simulink model "Grid_PV_three_phase"  (R2024a)
settings: Solver=VariableStepAuto  StartTime=0.0  StopTime=2.0  RelTol=1e-3
libraries: spsSeriesRLCBranchLib x12, spsIGBTDiodeLib x7, slpidlib x5, spsCurrentMeasurementLib x3, spsAlphaBetaZerotodq0Lib x3, simulink x2, spsabctoAlphaBetaZeroLib x2, spsThreePhaseVIMeasurementLib x2, spsPVArrayLib x1, spsDiodeLib x1, spsMeanLib x1, spsdq0toabcLib x1
settings Model: Creator=Ashmita  LastModifiedBy=Ashmita

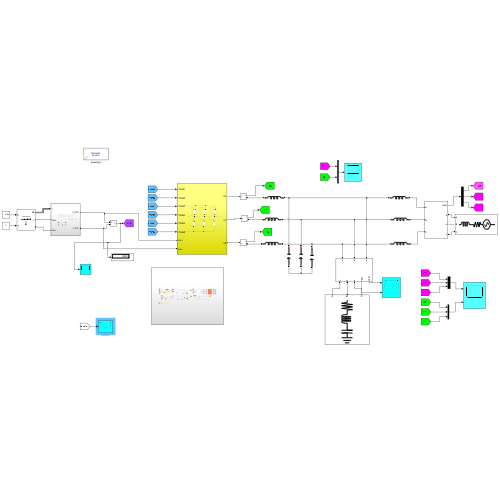
[thumbnail: Simulink's stored preview of the top-level diagram]
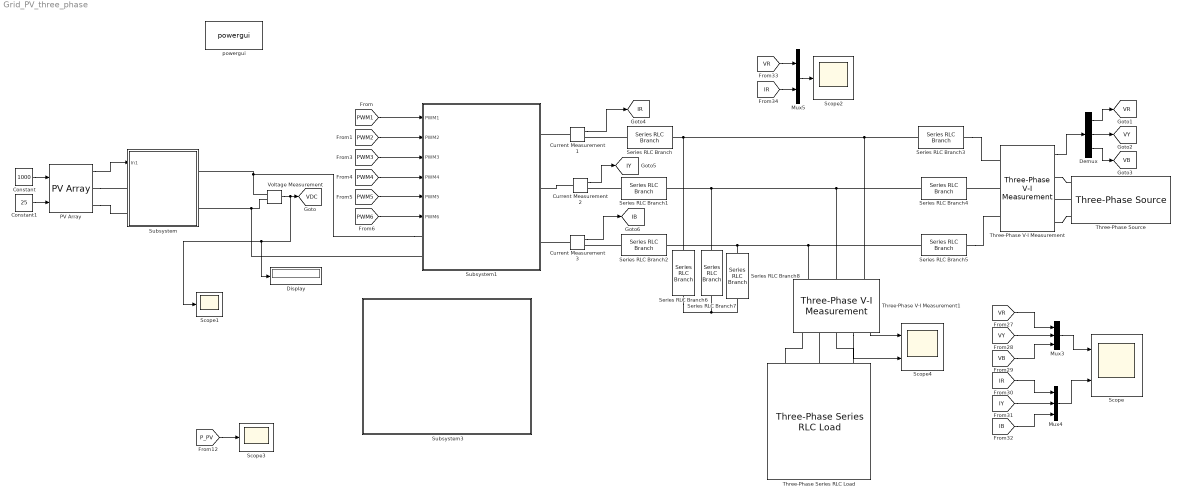
== system Grid_PV_three_phase ==
  Constant : Constant  Value=1000
  Constant1 : Constant  Value=25
  Current Measurement1 : spsCurrentMeasurementLib/Current Measurement  PhasorSimulation=off  OutputType=Complex  PSBequivalent=0
  Current Measurement2 : spsCurrentMeasurementLib/Current Measurement  PhasorSimulation=off  OutputType=Complex  PSBequivalent=0
  Current Measurement3 : spsCurrentMeasurementLib/Current Measurement  PhasorSimulation=off  OutputType=Complex  PSBequivalent=0
  Demux : Demux  Outputs=3
  Display : Display
  Mux3 : Mux  Inputs=3
  Mux4 : Mux  Inputs=3
  Mux5 : Mux  Inputs=2
  PV Array : spsPVArrayLib/PV Array  Npar=40  Nser=20  PlotType=array @ 1000 W/m2 & specified temperatures  S_vec="[ 1000  500  100 ]"  Temp_C_vec="[ 45 25  ]"  ModuleName=User-defined  PlotWhenSelected=off  Pm=213.15  Ncell=60  Voc=36.3  Isc=7.84  Vm=29  Im=7.35  beta_Voc_pc=-0.36099  alpha_Isc_pc=0.102  beta_Voc=-0.13104  alpha_Isc=0.0079968  IL=7.8654  I0=2.9273e-10  nI=0.98119  Rsh=313.0553  Rs=0.39381  RobustModel=off  RobustCellTemperature=313.3991  BAL=on  Tc=1e-6  Tfilter=5e-5
  Scope : Scope  NumInputPorts=2
  Scope1 : Scope
  Scope2 : Scope
  Scope3 : Scope
  Scope4 : Scope  NumInputPorts=2
  Series RLC Branch{,1..5} (6 alike) : spsSeriesRLCBranchLib/Series RLC Branch  LConnTagsString=__new0  RConnTagsString=__new0  BranchType=L  Resistance=1  Inductance=500e-6  SetiL0=off  InitialCurrent=0  Capacitance=1e-6  Setx0=off  InitialVoltage=0  Measurements=None
  Series RLC Branch6 : spsSeriesRLCBranchLib/Series RLC Branch  LConnTagsString=__new0  RConnTagsString=__new0  BranchType=C  Resistance=1  Inductance=500e-6  SetiL0=off  InitialCurrent=0  Capacitance=100e-6  Setx0=off  InitialVoltage=0  Measurements=None
  Series RLC Branch7 : spsSeriesRLCBranchLib/Series RLC Branch  LConnTagsString=__new0  RConnTagsString=__new0  BranchType=C  Resistance=1  Inductance=500e-6  SetiL0=off  InitialCurrent=0  Capacitance=100e-6  Setx0=off  InitialVoltage=0  Measurements=None
  Series RLC Branch8 : spsSeriesRLCBranchLib/Series RLC Branch  LConnTagsString=__new0  RConnTagsString=__new0  BranchType=C  Resistance=1  Inductance=500e-6  SetiL0=off  InitialCurrent=0  Capacitance=100e-6  Setx0=off  InitialVoltage=0  Measurements=None
  Subsystem : Subsystem
  Subsystem1 : Subsystem
  Subsystem3 : Subsystem
  Three-Phase Series RLC Load : spsThreePhaseSeriesRLCLoadLib/Three-Phase Series RLC Load  LConnTagsString=A|B|C  Configuration=Y (grounded)  NominalVoltage=1000  Vabc=[1e3 1e3 1e3]  Vabcp=[1e3 1e3 1e3]  NominalFrequency=60  UnbalancedPower=off  ActivePower=10e3  InductivePower=100  CapacitivePower=100  Pabc=[10e3 9e3 11e3]  QLabc=[100 90 110]  QCabc=[100 90 110]  Pabcp=[10e3 9e3 11e3]  QLabcp=[100 90 110]  QCabcp=[100 90 110]  Measurements=None  LoadType=constant Z
  Three-Phase V-I Measurement : spsThreePhaseVIMeasurementLib/Three-Phase V-I Measurement  VoltageMeasurement=phase-to-phase  SetLabelV=off  LabelV=Vabc  Vpu=off  VpuLL=off  CurrentMeasurement=no  SetLabelI=off  LabelI=Iabc  Ipu=off  Pbase=100e6  Vbase=500e3  OutputType=Complex  PhasorSimulation=off  PSBequivalent=0
  Three-Phase V-I Measurement1 : spsThreePhaseVIMeasurementLib/Three-Phase V-I Measurement  VoltageMeasurement=phase-to-phase  SetLabelV=off  LabelV=Vabc  Vpu=off  VpuLL=off  CurrentMeasurement=yes  SetLabelI=off  LabelI=Iabc  Ipu=off  Pbase=100e6  Vbase=500e3  OutputType=Complex  PhasorSimulation=off  PSBequivalent=0
  Three-Phase Source : spsThreePhaseSourceLib/Three-Phase Source  InternalConnection=Y  VoltagePhases=off  Voltage=415  PhaseAngle=0  Voltage_phases=[25e3 25e3 25e3]/sqrt(3)  PhaseAngles_phases=[0 -120 +120]  Frequency=50  NonIdealSource=on  SpecifyImpedance=off  Resistance=0.001e-3  Inductance=0.001e-9  ShortCircuitLevel=100e6  BaseVoltage=415  XRratio=7  BusType=swing  Pref=10e3  Qref=0  Prefabc=[10e3, 10e3, 10e3]  Qrefabc=[0, 0, 0]  Qmin=-inf  Qmax=inf
  Voltage Measurement : spsVoltageMeasurementLib/Voltage Measurement  PhasorSimulation=off  OutputType=Complex  PSBequivalent=0
  powergui : sps_lib/powergui  Priority=1  SimulationMode=Discrete  SampleTime=1e-6  frequency=60  Iterations=50  frequencyindice=50  Pbase=100e6  ErrMax=1e-4  UnitsV=kV  UnitsW=MW  buscounter=0  FunctionMessages=off  echomessages=off  EnableUseOfTLC=off  CurrentSourceSwitches=off  DisableSnubberDevices=off  DisableRonSwitches=off  DisableVfSwitches=off  DisplayEquations=off  AutomaticDiscreteSolvers=off  SolverType=Tustin/Backward Euler (TBE)  Interpol=off  ExternalGateDelay=off  methode=off  Ts=100  x0status=blocks  SPID=on  SwTol=0  HookPort=off  NonlinearTolerance=0  nMaxIteration=15  ContinueOnMaxIteration=off  RestoreLinks=warning  ResistiveCurrentMeasurement=off  Frange=[0:2:500]  Ylog=off  Xlog=on  ShowGrid=off  save=off  variable=ZData  structure=grid  ZoomFFT=on  StartTime=0.01  cycles=4  DisplayStyle=1  fundamental=50  FreqAxis=on  MaxFrequency=1000  frequencyindicesteady=1  RmsSteady=1  display=off
  tag scope: IB=global, IR=global, IY=global, VB=global, VDC=global, VR=global, VY=global
  wires:
  Constant1/1 -> PV Array/2
  PV Array/1 -> Subsystem/1(In1)
  Constant/1 -> PV Array/1
  Mux3/1 -> Scope/1
  [IR] -> Mux5/2
  [PWM6] -> Subsystem1/6("\tPWM6")
  [IR] -> Mux4/1
  [VR] -> Mux5/1
  [IY] -> Mux4/2
  [VB] -> Mux3/3
  [VY] -> Mux3/2
  [VR] -> Mux3/1
  [PWM3] -> Subsystem1/3("\tPWM3")
  [IB] -> Mux4/3
  Three-Phase V-I Measurement/1 -> Demux/1
  [PWM4] -> Subsystem1/4("\tPWM4")
  Current Measurement2/1 -> [IY]
  Mux4/1 -> Scope/2
  Demux/2 -> [VY]
  Demux/1 -> [VR]
  Demux/3 -> [VB]
  Current Measurement3/1 -> [IB]
  [PWM5] -> Subsystem1/5("\tPWM5")
  [PWM1] -> Subsystem1/1("\tPWM1 ")
  [PWM2] -> Subsystem1/2("\tPWM2")
  Current Measurement1/1 -> [IR]
  Mux5/1 -> Scope2/1
  Voltage Measurement/1 -> Display/1, Scope1/1, [VDC]
  Three-Phase V-I Measurement1/1 -> Scope4/1
  Three-Phase V-I Measurement1/2 -> Scope4/2
  [P_PV] -> Scope3/1
  connections:
  Voltage Measurement/LConn2 -- Subsystem1/LConn2 -- Subsystem/RConn2
  PV Array/RConn2 -- Subsystem/LConn2
  PV Array/RConn1 -- Subsystem/LConn1
  Subsystem1/LConn1 -- Subsystem/RConn1 -- Voltage Measurement/LConn1
  Series RLC Branch8/LConn1 -- Three-Phase V-I Measurement1/LConn3 -- Series RLC Branch5/LConn1 -- Series RLC Branch2/RConn1
  Series RLC Branch8/RConn1 -- Series RLC Branch6/RConn1 -- Series RLC Branch7/RConn1
  Series RLC Branch/RConn1 -- Three-Phase V-I Measurement1/LConn1 -- Series RLC Branch3/LConn1 -- Series RLC Branch6/LConn1
  Series RLC Branch1/RConn1 -- Three-Phase V-I Measurement1/LConn2 -- Series RLC Branch4/LConn1 -- Series RLC Branch7/LConn1
  Series RLC Branch2/LConn1 -- Current Measurement3/RConn1
  Series RLC Branch3/RConn1 -- Three-Phase V-I Measurement/LConn1
  Three-Phase Source/RConn2 -- Three-Phase V-I Measurement/RConn2
  Series RLC Branch/LConn1 -- Current Measurement1/RConn1
  Series RLC Branch1/LConn1 -- Current Measurement2/RConn1
  Current Measurement2/LConn1 -- Subsystem1/RConn2
  Three-Phase V-I Measurement/RConn1 -- Three-Phase Source/RConn1
  Series RLC Branch5/RConn1 -- Three-Phase V-I Measurement/LConn3
  Three-Phase V-I Measurement/LConn2 -- Series RLC Branch4/RConn1
  Current Measurement3/LConn1 -- Subsystem1/RConn3
  Three-Phase V-I Measurement/RConn3 -- Three-Phase Source/RConn3
  Current Measurement1/LConn1 -- Subsystem1/RConn1
  Three-Phase Series RLC Load/LConn1 -- Three-Phase V-I Measurement1/RConn3
  Three-Phase Series RLC Load/LConn2 -- Three-Phase V-I Measurement1/RConn2
  Three-Phase Series RLC Load/LConn3 -- Three-Phase V-I Measurement1/RConn1

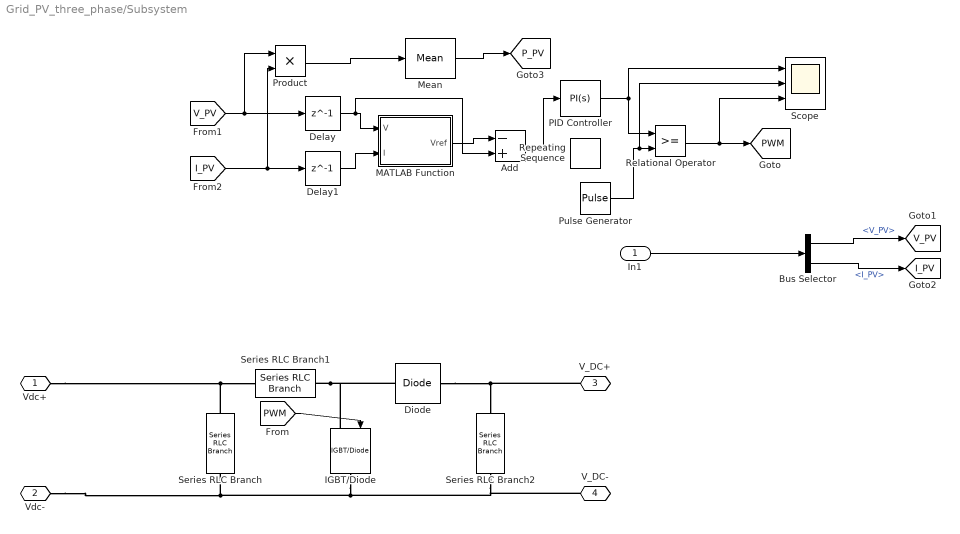
== system Grid_PV_three_phase/Subsystem ==
  In1 : Inport
  Add : Sum  Inputs=-+
  Bus Selector : BusSelector  OutputSignals=V_PV,I_PV
  Delay : Delay  DelayLength=1  InitialCondition=0
  Delay1 : Delay  DelayLength=1  InitialCondition=0
  Diode : spsDiodeLib/Diode  Ron=0.001  Lon=2.2e-3  Vf=0.7  IC=0  UseSnubber=0  Rs=10e3  Cs=inf  Measurements=off
  IGBT/Diode : spsIGBTDiodeLib/IGBT//Diode  Ron=.001  Rs=1e3  Cs=inf  Measurements=off
  MATLAB Function : MATLAB Function  TreatAsAtomicUnit=on
  Mean : spsMeanLib/Mean  Freq=60  Vinit=0  Ts=0
  PID Controller : slpidlib/PID Controller  Controller=PI  Form=Parallel  TimeDomain=Continuous-time  UseExternalTs=off  SampleTime=-1  IntegratorMethod=Forward Euler  FilterMethod=Forward Euler  ControllerParametersSource=internal  P=0.05  I=0.01  UseKiTs=off  D=0  UseExternalDerivativeSource=off  N=100  UseFilter=on  TunerSelectOption=Transfer Function Based (PID Tuner App)  InitialConditionSource=internal  InitialConditionForIntegrator=0  InitialConditionForFilter=0  DifferentiatorICPrevScaledInput=0  ExternalReset=none  TrackingMode=off  Kt=1  LimitOutput=on  SatLimitsSource=internal  UpperSaturationLimit=0.95  LowerSaturationLimit=0.00  LinearizeAsGain=on  AntiWindupMode=none  Kb=1  LimitIntegrator=off  UpperIntegratorSaturationLimit=inf  LowerIntegratorSaturationLimit=-inf  POutMin=[]  POutMax=[]  IOutMin=[]  IOutMax=[]  DOutMin=[]  DOutMax=[]  NOutMin=[]  NOutMax=[]  SumOutMin=[]  SumOutMax=[]  SaturationOutMin=[]  SaturationOutMax=[]  PParamMin=[]  PParamMax=[]  IParamMin=[]  IParamMax=[]  DParamMin=[]  DParamMax=[]  NParamMin=[]  NParamMax=[]  KbParamMin=[]  KbParamMax=[]  KtParamMin=[]  KtParamMax=[]  KbOutMin=[]  KbOutMax=[]  KtOutMin=[]  KtOutMax=[]  IntegratorOutMin=[]  IntegratorOutMax=[]  FilterOutMin=[]  FilterOutMax=[]  SumI1OutMin=[]  SumI1OutMax=[]  SumI2OutMin=[]  SumI2OutMax=[]  SumI3OutMin=[]  SumI3OutMax=[]  SumI4OutMin=[]  SumI4OutMax=[]  SumDOutMin=[]  SumDOutMax=[]  DifferentiatorOutMin=[]  DifferentiatorOutMax=[]  FilterDiffOutCoefMin=[]  FilterDiffOutCoefMax=[]  ReciprocalOutMin=[]  ReciprocalOutMax=[]  SumDenOutMin=[]  SumDenOutMax=[]  SumNumOutMin=[]  SumNumOutMax=[]  DivideOutMin=[]  DivideOutMax=[]  UdiffTsProdOutMin=[]  UdiffTsProdOutMax=[]  NTsProdOutMin=[]  NTsProdOutMax=[]  UintegralTsProdOutMin=[]  UintegralTsProdOutMax=[]  UngainTsProdOutMin=[]  UngainTsProdOutMax=[]  ClampingZeroOutDataTypeStr=Inherit: Inherit via back propagation  ClampingZeroOutMin=[]  ClampingZeroOutMax=[]  FilterDenConstantOutDataTypeStr=Inherit: Inherit via back propagation  FilterDenConstantOutMin=[]  FilterDenConstantOutMax=[]  PCopyOutDataTypeStr=Inherit: Inherit via back propagation  PCopyOutMin=[]  PCopyOutMax=[]  NCopyOutDataTypeStr=Inherit: Inherit via back propagation  NCopyOutMin=[]  NCopyOutMax=[]  IntegratorContinuousStateAttributes=''  IntegratorStateMustResolveToSignalObject=off  IntegratorRTWStateStorageClass=Auto  FilterContinuousStateAttributes=''  FilterStateMustResolveToSignalObject=off  FilterRTWStateStorageClass=Auto  ParallelPVariant=InternalParameters  IdealPVariant=Disabled  IVariant=InternalParameters  DVariant=Disabled  IntegratorVariant=Continuous  SatVariant=Enabled  AWVariant=Passthrough  PCopyVariant=Disabled  TRVariant=Disabled  FdbkBlocksVariant=Forward  IdealPFdbkVariant=Disabled  SatFdbkVariant=Disabled  DerivativeFilterVariant=Disabled  NVariant=Disabled  NCopyVariant=Disabled_SignalSpec  FilterICVariant=Disabled  IntegratorICVariant=InternalICs  ExternalResetVariant=Disabled  TRSumVariant=Passthrough  SumFdbkVariant=Disabled  SumVariant=Sum_PI  TsampFilterVariant=InternalTs  TsampNgainVariant=Passthrough  TsampIntegralVariant=Disabled_SignalSpec  ExternalSaturationOutDataTypeStr=Inherit: Same as second input  DerivativeSourceVariant=Disabled
  Product : Product
  Pulse Generator : DiscretePulseGenerator  PulseType=Time based  Period=1/500000  PulseWidth=90
  Relational Operator : RelationalOperator  OutDataTypeStr=boolean  RndMeth=Simplest  InputSameDT=off
  Repeating Sequence : simulink/Sources/Repeating Sequence  rep_seq_t=[0 1/5000]  rep_seq_y=[0 1]
  Scope : Scope  NumInputPorts=3
  Series RLC Branch : spsSeriesRLCBranchLib/Series RLC Branch  LConnTagsString=__new0  RConnTagsString=__new0  BranchType=C  Resistance=1e-6  Inductance=1e-3  SetiL0=off  InitialCurrent=0  Capacitance=1000e-6  Setx0=off  InitialVoltage=0  Measurements=None
  Series RLC Branch1 : spsSeriesRLCBranchLib/Series RLC Branch  LConnTagsString=__new0  RConnTagsString=__new0  BranchType=L  Resistance=1  Inductance=1.45e-3  SetiL0=off  InitialCurrent=0  Capacitance=1e-6  Setx0=off  InitialVoltage=0  Measurements=None
  Series RLC Branch2 : spsSeriesRLCBranchLib/Series RLC Branch  LConnTagsString=__new0  RConnTagsString=__new0  BranchType=C  Resistance=1  Inductance=1e-3  SetiL0=off  InitialCurrent=0  Capacitance=3227e-6  Setx0=off  InitialVoltage=0  Measurements=None
  Vdc+ : PMIOPort  Side=Left
  V_DC+ : PMIOPort  Port=3  Side=Right
  V_DC- : PMIOPort  Port=4  Side=Right
  Vdc- : PMIOPort  Port=2  Side=Left
  tag scope: I_PV=global, PWM=global, P_PV=global, V_PV=global
  wires:
  [V_PV] -> Product/1, Delay/1
  [I_PV] -> Product/2, Delay1/1
  Mean/1 -> [P_PV]
  Add/1 -> PID Controller/1
  Delay/1 -> Add/2, MATLAB Function/1(V)
  Product/1 -> Mean/1
  Bus Selector/1 -> [V_PV]  "<V_PV>"
  MATLAB Function/1(Vref) -> Add/1
  PID Controller/1 -> Relational Operator/1, Scope/1
  Relational Operator/1 -> Scope/3, [PWM]
  Delay1/1 -> MATLAB Function/2(I)
  Bus Selector/2 -> [I_PV]  "<I_PV>"
  [PWM] -> IGBT/Diode/1
  In1/1 -> Bus Selector/1
  Pulse Generator/1 -> Scope/2, Relational Operator/2
  connections:
  Diode/RConn1 -- V_DC+/RConn1 -- Series RLC Branch2/LConn1
  Series RLC Branch1/LConn1 -- IGBT/Diode/LConn1 -- Diode/LConn1
  IGBT/Diode/RConn1 -- V_DC-/RConn1 -- Series RLC Branch2/RConn1 -- Vdc-/RConn1 -- Series RLC Branch/RConn1
  Series RLC Branch/LConn1 -- Vdc+/RConn1 -- Series RLC Branch1/RConn1

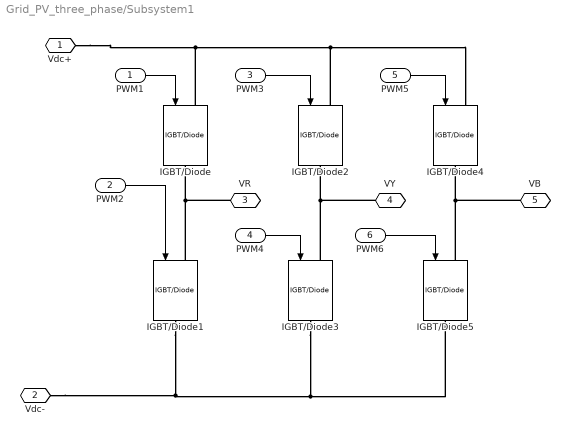
== system Grid_PV_three_phase/Subsystem1 ==
  "\tPWM1 " : Inport
  "\tPWM2" : Inport  Port=2
  "\tPWM3" : Inport  Port=3
  "\tPWM4" : Inport  Port=4
  "\tPWM5" : Inport  Port=5
  "\tPWM6" : Inport  Port=6
  IGBT/Diode{,1..5} (6 alike) : spsIGBTDiodeLib/IGBT//Diode  Ron=1e-3  Rs=1e5  Cs=inf  Measurements=off
  Vdc+ : PMIOPort  Side=Left
  Vdc- : PMIOPort  Port=2  Side=Left
  VR : PMIOPort  Port=3  Side=Right
  VY : PMIOPort  Port=4  Side=Right
  VB : PMIOPort  Port=5  Side=Right
  wires:
  "\tPWM4"/1 -> IGBT/Diode3/1
  "\tPWM5"/1 -> IGBT/Diode4/1
  "\tPWM2"/1 -> IGBT/Diode1/1
  "\tPWM1 "/1 -> IGBT/Diode/1
  "\tPWM6"/1 -> IGBT/Diode5/1
  "\tPWM3"/1 -> IGBT/Diode2/1
  connections:
  IGBT/Diode5/LConn1 -- VB/RConn1 -- IGBT/Diode4/RConn1
  IGBT/Diode/LConn1 -- Vdc+/RConn1 -- IGBT/Diode2/LConn1 -- IGBT/Diode4/LConn1
  IGBT/Diode1/LConn1 -- VR/RConn1 -- IGBT/Diode/RConn1
  IGBT/Diode1/RConn1 -- IGBT/Diode3/RConn1 -- IGBT/Diode5/RConn1 -- Vdc-/RConn1
  IGBT/Diode3/LConn1 -- VY/RConn1 -- IGBT/Diode2/RConn1

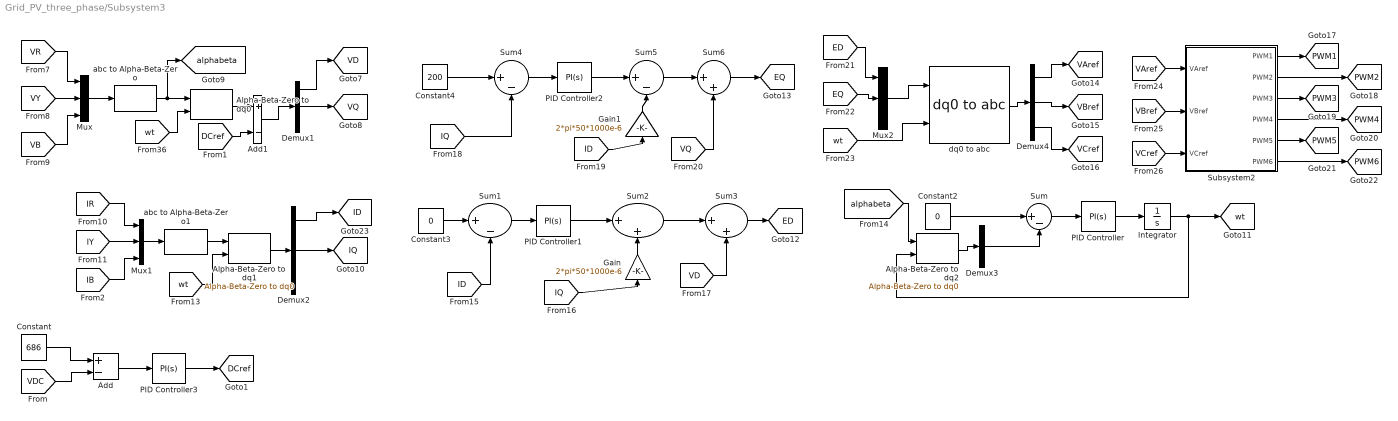
== system Grid_PV_three_phase/Subsystem3 ==
  Add : Sum  Inputs=+-
  Add1 : Sum  Inputs=+-
  Alpha-Beta-Zero to dq0 : spsAlphaBetaZerotodq0Lib/Alpha-Beta-Zero to dq0  Alignment=90 degrees behind phase A axis
  Alpha-Beta-Zero to dq1 : spsAlphaBetaZerotodq0Lib/Alpha-Beta-Zero to dq0  Alignment=90 degrees behind phase A axis
  Alpha-Beta-Zero to dq2 : spsAlphaBetaZerotodq0Lib/Alpha-Beta-Zero to dq0  Alignment=90 degrees behind phase A axis
  Constant : Constant  Value=686
  Constant2 : Constant  Value=0
  Constant3 : Constant  Value=0
  Constant4 : Constant  Value=200
  Demux{1..4} (4 alike) : Demux  Outputs=3
  Gain : Gain  Gain=2*pi*50*1000e-6
  Gain1 : Gain  Gain=2*pi*50*1000e-6
  Integrator : Integrator
  Mux : Mux  Inputs=3
  Mux1 : Mux  Inputs=3
  Mux2 : Mux  Inputs=3
  PID Controller : slpidlib/PID Controller  Controller=PI  Form=Parallel  TimeDomain=Continuous-time  UseExternalTs=off  SampleTime=-1  IntegratorMethod=Forward Euler  FilterMethod=Forward Euler  ControllerParametersSource=internal  P=10  I=50000  UseKiTs=off  D=0  UseExternalDerivativeSource=off  N=100  UseFilter=on  TunerSelectOption=Transfer Function Based (PID Tuner App)  InitialConditionSource=internal  InitialConditionForIntegrator=0  InitialConditionForFilter=0  DifferentiatorICPrevScaledInput=0  ExternalReset=none  TrackingMode=off  Kt=1  LimitOutput=off  SatLimitsSource=internal  UpperSaturationLimit=inf  LowerSaturationLimit=-inf  LinearizeAsGain=on  AntiWindupMode=none  Kb=1  LimitIntegrator=off  UpperIntegratorSaturationLimit=inf  LowerIntegratorSaturationLimit=-inf  POutMin=[]  POutMax=[]  IOutMin=[]  IOutMax=[]  DOutMin=[]  DOutMax=[]  NOutMin=[]  NOutMax=[]  SumOutMin=[]  SumOutMax=[]  SaturationOutMin=[]  SaturationOutMax=[]  PParamMin=[]  PParamMax=[]  IParamMin=[]  IParamMax=[]  DParamMin=[]  DParamMax=[]  NParamMin=[]  NParamMax=[]  KbParamMin=[]  KbParamMax=[]  KtParamMin=[]  KtParamMax=[]  KbOutMin=[]  KbOutMax=[]  KtOutMin=[]  KtOutMax=[]  IntegratorOutMin=[]  IntegratorOutMax=[]  FilterOutMin=[]  FilterOutMax=[]  SumI1OutMin=[]  SumI1OutMax=[]  SumI2OutMin=[]  SumI2OutMax=[]  SumI3OutMin=[]  SumI3OutMax=[]  SumI4OutMin=[]  SumI4OutMax=[]  SumDOutMin=[]  SumDOutMax=[]  DifferentiatorOutMin=[]  DifferentiatorOutMax=[]  FilterDiffOutCoefMin=[]  FilterDiffOutCoefMax=[]  ReciprocalOutMin=[]  ReciprocalOutMax=[]  SumDenOutMin=[]  SumDenOutMax=[]  SumNumOutMin=[]  SumNumOutMax=[]  DivideOutMin=[]  DivideOutMax=[]  UdiffTsProdOutMin=[]  UdiffTsProdOutMax=[]  NTsProdOutMin=[]  NTsProdOutMax=[]  UintegralTsProdOutMin=[]  UintegralTsProdOutMax=[]  UngainTsProdOutMin=[]  UngainTsProdOutMax=[]  ClampingZeroOutDataTypeStr=Inherit: Inherit via back propagation  ClampingZeroOutMin=[]  ClampingZeroOutMax=[]  FilterDenConstantOutDataTypeStr=Inherit: Inherit via back propagation  FilterDenConstantOutMin=[]  FilterDenConstantOutMax=[]  PCopyOutDataTypeStr=Inherit: Inherit via back propagation  PCopyOutMin=[]  PCopyOutMax=[]  NCopyOutDataTypeStr=Inherit: Inherit via back propagation  NCopyOutMin=[]  NCopyOutMax=[]  IntegratorContinuousStateAttributes=''  IntegratorStateMustResolveToSignalObject=off  IntegratorRTWStateStorageClass=Auto  FilterContinuousStateAttributes=''  FilterStateMustResolveToSignalObject=off  FilterRTWStateStorageClass=Auto  ParallelPVariant=InternalParameters  IdealPVariant=Disabled  IVariant=InternalParameters  DVariant=Disabled  IntegratorVariant=Continuous  SatVariant=Disabled  AWVariant=Passthrough  PCopyVariant=Disabled  TRVariant=Disabled  FdbkBlocksVariant=Forward  IdealPFdbkVariant=Disabled  SatFdbkVariant=Disabled  DerivativeFilterVariant=Disabled  NVariant=Disabled  NCopyVariant=Disabled_SignalSpec  FilterICVariant=Disabled  IntegratorICVariant=InternalICs  ExternalResetVariant=Disabled  TRSumVariant=Passthrough  SumFdbkVariant=Disabled  SumVariant=Sum_PI  TsampFilterVariant=InternalTs  TsampNgainVariant=Passthrough  TsampIntegralVariant=Disabled_SignalSpec  ExternalSaturationOutDataTypeStr=Inherit: Same as second input  DerivativeSourceVariant=Disabled
  PID Controller1 : slpidlib/PID Controller  Controller=PI  Form=Parallel  TimeDomain=Continuous-time  UseExternalTs=off  SampleTime=-1  IntegratorMethod=Forward Euler  FilterMethod=Forward Euler  ControllerParametersSource=internal  P=5  I=5000  UseKiTs=off  D=0  UseExternalDerivativeSource=off  N=100  UseFilter=on  TunerSelectOption=Transfer Function Based (PID Tuner App)  InitialConditionSource=internal  InitialConditionForIntegrator=0  InitialConditionForFilter=0  DifferentiatorICPrevScaledInput=0  ExternalReset=none  TrackingMode=off  Kt=1  LimitOutput=off  SatLimitsSource=internal  UpperSaturationLimit=inf  LowerSaturationLimit=-inf  LinearizeAsGain=on  AntiWindupMode=none  Kb=1  LimitIntegrator=off  UpperIntegratorSaturationLimit=inf  LowerIntegratorSaturationLimit=-inf  POutMin=[]  POutMax=[]  IOutMin=[]  IOutMax=[]  DOutMin=[]  DOutMax=[]  NOutMin=[]  NOutMax=[]  SumOutMin=[]  SumOutMax=[]  SaturationOutMin=[]  SaturationOutMax=[]  PParamMin=[]  PParamMax=[]  IParamMin=[]  IParamMax=[]  DParamMin=[]  DParamMax=[]  NParamMin=[]  NParamMax=[]  KbParamMin=[]  KbParamMax=[]  KtParamMin=[]  KtParamMax=[]  KbOutMin=[]  KbOutMax=[]  KtOutMin=[]  KtOutMax=[]  IntegratorOutMin=[]  IntegratorOutMax=[]  FilterOutMin=[]  FilterOutMax=[]  SumI1OutMin=[]  SumI1OutMax=[]  SumI2OutMin=[]  SumI2OutMax=[]  SumI3OutMin=[]  SumI3OutMax=[]  SumI4OutMin=[]  SumI4OutMax=[]  SumDOutMin=[]  SumDOutMax=[]  DifferentiatorOutMin=[]  DifferentiatorOutMax=[]  FilterDiffOutCoefMin=[]  FilterDiffOutCoefMax=[]  ReciprocalOutMin=[]  ReciprocalOutMax=[]  SumDenOutMin=[]  SumDenOutMax=[]  SumNumOutMin=[]  SumNumOutMax=[]  DivideOutMin=[]  DivideOutMax=[]  UdiffTsProdOutMin=[]  UdiffTsProdOutMax=[]  NTsProdOutMin=[]  NTsProdOutMax=[]  UintegralTsProdOutMin=[]  UintegralTsProdOutMax=[]  UngainTsProdOutMin=[]  UngainTsProdOutMax=[]  ClampingZeroOutDataTypeStr=Inherit: Inherit via back propagation  ClampingZeroOutMin=[]  ClampingZeroOutMax=[]  FilterDenConstantOutDataTypeStr=Inherit: Inherit via back propagation  FilterDenConstantOutMin=[]  FilterDenConstantOutMax=[]  PCopyOutDataTypeStr=Inherit: Inherit via back propagation  PCopyOutMin=[]  PCopyOutMax=[]  NCopyOutDataTypeStr=Inherit: Inherit via back propagation  NCopyOutMin=[]  NCopyOutMax=[]  IntegratorContinuousStateAttributes=''  IntegratorStateMustResolveToSignalObject=off  IntegratorRTWStateStorageClass=Auto  FilterContinuousStateAttributes=''  FilterStateMustResolveToSignalObject=off  FilterRTWStateStorageClass=Auto  ParallelPVariant=InternalParameters  IdealPVariant=Disabled  IVariant=InternalParameters  DVariant=Disabled  IntegratorVariant=Continuous  SatVariant=Disabled  AWVariant=Passthrough  PCopyVariant=Disabled  TRVariant=Disabled  FdbkBlocksVariant=Forward  IdealPFdbkVariant=Disabled  SatFdbkVariant=Disabled  DerivativeFilterVariant=Disabled  NVariant=Disabled  NCopyVariant=Disabled_SignalSpec  FilterICVariant=Disabled  IntegratorICVariant=InternalICs  ExternalResetVariant=Disabled  TRSumVariant=Passthrough  SumFdbkVariant=Disabled  SumVariant=Sum_PI  TsampFilterVariant=InternalTs  TsampNgainVariant=Passthrough  TsampIntegralVariant=Disabled_SignalSpec  ExternalSaturationOutDataTypeStr=Inherit: Same as second input  DerivativeSourceVariant=Disabled
  PID Controller2 : slpidlib/PID Controller  Controller=PI  Form=Parallel  TimeDomain=Continuous-time  UseExternalTs=off  SampleTime=-1  IntegratorMethod=Forward Euler  FilterMethod=Forward Euler  ControllerParametersSource=internal  P=5  I=5000  UseKiTs=off  D=0  UseExternalDerivativeSource=off  N=100  UseFilter=on  TunerSelectOption=Transfer Function Based (PID Tuner App)  InitialConditionSource=internal  InitialConditionForIntegrator=0  InitialConditionForFilter=0  DifferentiatorICPrevScaledInput=0  ExternalReset=none  TrackingMode=off  Kt=1  LimitOutput=off  SatLimitsSource=internal  UpperSaturationLimit=inf  LowerSaturationLimit=-inf  LinearizeAsGain=on  AntiWindupMode=none  Kb=1  LimitIntegrator=off  UpperIntegratorSaturationLimit=inf  LowerIntegratorSaturationLimit=-inf  POutMin=[]  POutMax=[]  IOutMin=[]  IOutMax=[]  DOutMin=[]  DOutMax=[]  NOutMin=[]  NOutMax=[]  SumOutMin=[]  SumOutMax=[]  SaturationOutMin=[]  SaturationOutMax=[]  PParamMin=[]  PParamMax=[]  IParamMin=[]  IParamMax=[]  DParamMin=[]  DParamMax=[]  NParamMin=[]  NParamMax=[]  KbParamMin=[]  KbParamMax=[]  KtParamMin=[]  KtParamMax=[]  KbOutMin=[]  KbOutMax=[]  KtOutMin=[]  KtOutMax=[]  IntegratorOutMin=[]  IntegratorOutMax=[]  FilterOutMin=[]  FilterOutMax=[]  SumI1OutMin=[]  SumI1OutMax=[]  SumI2OutMin=[]  SumI2OutMax=[]  SumI3OutMin=[]  SumI3OutMax=[]  SumI4OutMin=[]  SumI4OutMax=[]  SumDOutMin=[]  SumDOutMax=[]  DifferentiatorOutMin=[]  DifferentiatorOutMax=[]  FilterDiffOutCoefMin=[]  FilterDiffOutCoefMax=[]  ReciprocalOutMin=[]  ReciprocalOutMax=[]  SumDenOutMin=[]  SumDenOutMax=[]  SumNumOutMin=[]  SumNumOutMax=[]  DivideOutMin=[]  DivideOutMax=[]  UdiffTsProdOutMin=[]  UdiffTsProdOutMax=[]  NTsProdOutMin=[]  NTsProdOutMax=[]  UintegralTsProdOutMin=[]  UintegralTsProdOutMax=[]  UngainTsProdOutMin=[]  UngainTsProdOutMax=[]  ClampingZeroOutDataTypeStr=Inherit: Inherit via back propagation  ClampingZeroOutMin=[]  ClampingZeroOutMax=[]  FilterDenConstantOutDataTypeStr=Inherit: Inherit via back propagation  FilterDenConstantOutMin=[]  FilterDenConstantOutMax=[]  PCopyOutDataTypeStr=Inherit: Inherit via back propagation  PCopyOutMin=[]  PCopyOutMax=[]  NCopyOutDataTypeStr=Inherit: Inherit via back propagation  NCopyOutMin=[]  NCopyOutMax=[]  IntegratorContinuousStateAttributes=''  IntegratorStateMustResolveToSignalObject=off  IntegratorRTWStateStorageClass=Auto  FilterContinuousStateAttributes=''  FilterStateMustResolveToSignalObject=off  FilterRTWStateStorageClass=Auto  ParallelPVariant=InternalParameters  IdealPVariant=Disabled  IVariant=InternalParameters  DVariant=Disabled  IntegratorVariant=Continuous  SatVariant=Disabled  AWVariant=Passthrough  PCopyVariant=Disabled  TRVariant=Disabled  FdbkBlocksVariant=Forward  IdealPFdbkVariant=Disabled  SatFdbkVariant=Disabled  DerivativeFilterVariant=Disabled  NVariant=Disabled  NCopyVariant=Disabled_SignalSpec  FilterICVariant=Disabled  IntegratorICVariant=InternalICs  ExternalResetVariant=Disabled  TRSumVariant=Passthrough  SumFdbkVariant=Disabled  SumVariant=Sum_PI  TsampFilterVariant=InternalTs  TsampNgainVariant=Passthrough  TsampIntegralVariant=Disabled_SignalSpec  ExternalSaturationOutDataTypeStr=Inherit: Same as second input  DerivativeSourceVariant=Disabled
  PID Controller3 : slpidlib/PID Controller  Controller=PI  Form=Parallel  TimeDomain=Continuous-time  UseExternalTs=off  SampleTime=-1  IntegratorMethod=Forward Euler  FilterMethod=Forward Euler  ControllerParametersSource=internal  P=1  I=1  UseKiTs=off  D=0  UseExternalDerivativeSource=off  N=100  UseFilter=on  TunerSelectOption=Transfer Function Based (PID Tuner App)  InitialConditionSource=internal  InitialConditionForIntegrator=0  InitialConditionForFilter=0  DifferentiatorICPrevScaledInput=0  ExternalReset=none  TrackingMode=off  Kt=1  LimitOutput=off  SatLimitsSource=internal  UpperSaturationLimit=inf  LowerSaturationLimit=-inf  LinearizeAsGain=on  AntiWindupMode=none  Kb=1  LimitIntegrator=off  UpperIntegratorSaturationLimit=inf  LowerIntegratorSaturationLimit=-inf  POutMin=[]  POutMax=[]  IOutMin=[]  IOutMax=[]  DOutMin=[]  DOutMax=[]  NOutMin=[]  NOutMax=[]  SumOutMin=[]  SumOutMax=[]  SaturationOutMin=[]  SaturationOutMax=[]  PParamMin=[]  PParamMax=[]  IParamMin=[]  IParamMax=[]  DParamMin=[]  DParamMax=[]  NParamMin=[]  NParamMax=[]  KbParamMin=[]  KbParamMax=[]  KtParamMin=[]  KtParamMax=[]  KbOutMin=[]  KbOutMax=[]  KtOutMin=[]  KtOutMax=[]  IntegratorOutMin=[]  IntegratorOutMax=[]  FilterOutMin=[]  FilterOutMax=[]  SumI1OutMin=[]  SumI1OutMax=[]  SumI2OutMin=[]  SumI2OutMax=[]  SumI3OutMin=[]  SumI3OutMax=[]  SumI4OutMin=[]  SumI4OutMax=[]  SumDOutMin=[]  SumDOutMax=[]  DifferentiatorOutMin=[]  DifferentiatorOutMax=[]  FilterDiffOutCoefMin=[]  FilterDiffOutCoefMax=[]  ReciprocalOutMin=[]  ReciprocalOutMax=[]  SumDenOutMin=[]  SumDenOutMax=[]  SumNumOutMin=[]  SumNumOutMax=[]  DivideOutMin=[]  DivideOutMax=[]  UdiffTsProdOutMin=[]  UdiffTsProdOutMax=[]  NTsProdOutMin=[]  NTsProdOutMax=[]  UintegralTsProdOutMin=[]  UintegralTsProdOutMax=[]  UngainTsProdOutMin=[]  UngainTsProdOutMax=[]  ClampingZeroOutDataTypeStr=Inherit: Inherit via back propagation  ClampingZeroOutMin=[]  ClampingZeroOutMax=[]  FilterDenConstantOutDataTypeStr=Inherit: Inherit via back propagation  FilterDenConstantOutMin=[]  FilterDenConstantOutMax=[]  PCopyOutDataTypeStr=Inherit: Inherit via back propagation  PCopyOutMin=[]  PCopyOutMax=[]  NCopyOutDataTypeStr=Inherit: Inherit via back propagation  NCopyOutMin=[]  NCopyOutMax=[]  IntegratorContinuousStateAttributes=''  IntegratorStateMustResolveToSignalObject=off  IntegratorRTWStateStorageClass=Auto  FilterContinuousStateAttributes=''  FilterStateMustResolveToSignalObject=off  FilterRTWStateStorageClass=Auto  ParallelPVariant=InternalParameters  IdealPVariant=Disabled  IVariant=InternalParameters  DVariant=Disabled  IntegratorVariant=Continuous  SatVariant=Disabled  AWVariant=Passthrough  PCopyVariant=Disabled  TRVariant=Disabled  FdbkBlocksVariant=Forward  IdealPFdbkVariant=Disabled  SatFdbkVariant=Disabled  DerivativeFilterVariant=Disabled  NVariant=Disabled  NCopyVariant=Disabled_SignalSpec  FilterICVariant=Disabled  IntegratorICVariant=InternalICs  ExternalResetVariant=Disabled  TRSumVariant=Passthrough  SumFdbkVariant=Disabled  SumVariant=Sum_PI  TsampFilterVariant=InternalTs  TsampNgainVariant=Passthrough  TsampIntegralVariant=Disabled_SignalSpec  ExternalSaturationOutDataTypeStr=Inherit: Same as second input  DerivativeSourceVariant=Disabled
  Subsystem2 : Subsystem
  Sum{,1,4..5} (4 alike) : Sum  Inputs=|+-
  Sum2 : Sum  Inputs=|++
  Sum3 : Sum  Inputs=|++
  Sum6 : Sum  Inputs=|++
  abc to Alpha-Beta-Zero : spsabctoAlphaBetaZeroLib/abc to Alpha-Beta-Zero
  abc to Alpha-Beta-Zero1 : spsabctoAlphaBetaZeroLib/abc to Alpha-Beta-Zero
  dq0 to abc : spsdq0toabcLib/dq0 to abc  Alignment=90 degrees behind phase A axis
  tag scope: DCref=global, ED=global, EQ=global, ID=global, IQ=global, PWM1=global, PWM2=global, PWM3=global, PWM4=global, PWM5=global, PWM6=global, VAref=global, VBref=global, VCref=global, VD=global, VQ=global, alphabeta=global, wt=global
  wires:
  [IB] -> Mux1/3
  Sum/1 -> PID Controller/1
  Sum6/1 -> [EQ]
  Demux2/2 -> [IQ]
  [ED] -> Mux2/1
  Subsystem2/4(PWM4) -> [PWM4]
  Subsystem2/1(PWM1) -> [PWM1]
  Sum3/1 -> [ED]
  [IY] -> Mux1/2
  Constant2/1 -> Sum/1
  Subsystem2/6(PWM6) -> [PWM6]
  Demux2/1 -> [ID]
  Sum1/1 -> PID Controller1/1
  Mux2/1 -> dq0 to abc/1
  [VCref] -> Subsystem2/3(VCref)
  PID Controller1/1 -> Sum2/1
  [alphabeta] -> Alpha-Beta-Zero to dq2/1
  Constant3/1 -> Sum1/1
  abc to Alpha-Beta-Zero1/1 -> Alpha-Beta-Zero to dq1/1
  [VR] -> Mux/1
  [EQ] -> Mux2/2
  Gain/1 -> Sum2/2
  Gain1/1 -> Sum5/2
  Sum2/1 -> Sum3/1
  [IR] -> Mux1/1
  Mux1/1 -> abc to Alpha-Beta-Zero1/1
  Alpha-Beta-Zero to dq2/1 -> Demux3/1
  [VB] -> Mux/3
  [VBref] -> Subsystem2/2(VBref)
  Subsystem2/2(PWM2) -> [PWM2]
  Alpha-Beta-Zero to dq1/1 -> Demux2/1
  [wt] -> Alpha-Beta-Zero to dq1/2
  Subsystem2/5(PWM5) -> [PWM5]
  Demux4/1 -> [VAref]
  Demux4/2 -> [VBref]
  Demux3/2 -> Sum/2
  abc to Alpha-Beta-Zero/1 -> [alphabeta], Alpha-Beta-Zero to dq0/1
  [VAref] -> Subsystem2/1(VAref)
  [wt] -> Alpha-Beta-Zero to dq0/2
  [wt] -> dq0 to abc/2
  Sum4/1 -> PID Controller2/1
  [IQ] -> Gain/1
  [ID] -> Sum1/2
  Constant4/1 -> Sum4/1
  [VD] -> Sum3/2
  Demux4/3 -> [VCref]
  dq0 to abc/1 -> Demux4/1
  PID Controller/1 -> Integrator/1
  Integrator/1 -> [wt], Alpha-Beta-Zero to dq2/2
  [VQ] -> Sum6/2
  [IQ] -> Sum4/2
  Mux/1 -> abc to Alpha-Beta-Zero/1
  Sum5/1 -> Sum6/1
  PID Controller2/1 -> Sum5/1
  Subsystem2/3(PWM3) -> [PWM3]
  [VY] -> Mux/2
  [ID] -> Gain1/1
  Demux1/2 -> [VQ]
  Demux1/1 -> [VD]
  Constant/1 -> Add/1
  Add/1 -> PID Controller3/1
  [VDC] -> Add/2
  Alpha-Beta-Zero to dq0/1 -> Add1/1
  Add1/1 -> Demux1/1
  PID Controller3/1 -> [DCref]
  [DCref] -> Add1/2

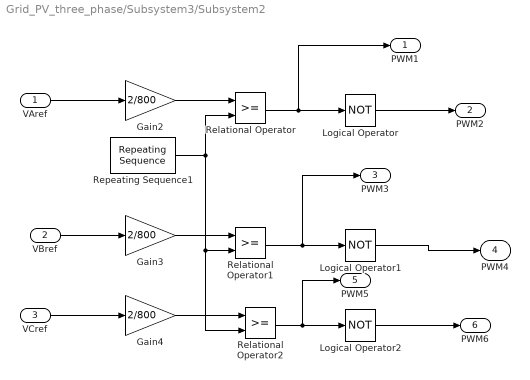
== system Grid_PV_three_phase/Subsystem3/Subsystem2 ==
  VAref : Inport
  VBref : Inport  Port=2
  VCref : Inport  Port=3
  Gain2 : Gain  Gain=2/800
  Gain3 : Gain  Gain=2/800
  Gain4 : Gain  Gain=2/800
  Logical Operator : Logic  Operator=NOT  AllPortsSameDT=off  OutDataTypeStr=boolean
  Logical Operator1 : Logic  Operator=NOT  AllPortsSameDT=off  OutDataTypeStr=boolean
  Logical Operator2 : Logic  Operator=NOT  AllPortsSameDT=off  OutDataTypeStr=boolean
  Relational Operator : RelationalOperator  OutDataTypeStr=boolean  RndMeth=Simplest  InputSameDT=off
  Relational Operator1 : RelationalOperator  OutDataTypeStr=boolean  RndMeth=Simplest  InputSameDT=off
  Relational Operator2 : RelationalOperator  OutDataTypeStr=boolean  RndMeth=Simplest  InputSameDT=off
  Repeating Sequence1 : simulink/Sources/Repeating Sequence  rep_seq_t=[0 0.00005 0.0001]  rep_seq_y=[-1 1 -1]
  PWM1 : Outport  VectorParamsAs1DForOutWhenUnconnected=off
  PWM2 : Outport  Port=2  VectorParamsAs1DForOutWhenUnconnected=off
  PWM3 : Outport  Port=3  VectorParamsAs1DForOutWhenUnconnected=off
  PWM4 : Outport  Port=4  VectorParamsAs1DForOutWhenUnconnected=off
  PWM5 : Outport  Port=5  VectorParamsAs1DForOutWhenUnconnected=off
  PWM6 : Outport  Port=6  VectorParamsAs1DForOutWhenUnconnected=off
  wires:
  Relational Operator2/1 -> PWM5/1, Logical Operator2/1
  Gain2/1 -> Relational Operator/1
  VCref/1 -> Gain4/1
  Gain4/1 -> Relational Operator2/1
  Relational Operator/1 -> PWM1/1, Logical Operator/1
  Repeating Sequence1/1 -> Relational Operator2/2, Relational Operator1/2, Relational Operator/2
  Logical Operator2/1 -> PWM6/1
  VAref/1 -> Gain2/1
  Relational Operator1/1 -> PWM3/1, Logical Operator1/1
  Logical Operator/1 -> PWM2/1
  Logical Operator1/1 -> PWM4/1
  Gain3/1 -> Relational Operator1/1
  VBref/1 -> Gain3/1

== matlab function Grid_PV_three_phase/Subsystem/MATLAB Function ==
  data: V input; Vref output; I input
function Vref = RefGen(V,I)
 
Vrefmax=900;
Vrefmin=0;
Vrefinit=300;
deltaVref=1;
persistent Vold Pold Vrefold;
 
dataType = 'double';
 
if isempty(Vold)
    Vold=0;
    Pold=0;
    Vrefold=Vrefinit;
end
 
P=V*I;
dV=V-Vold;
dP=P-Pold;
 
if dP~=0
    if dP<0
        if dV<0
            Vref=Vrefold+deltaVref;
        else
            Vref=Vrefold-deltaVref;
        end
    else
        if dV<0
            Vref=Vrefold-deltaVref;
        else
            Vref=Vrefold+deltaVref;
        end
    end
else
    Vref=Vrefold;
end
 
if Vref>=Vrefmax | Vref<= Vrefmin
    Vref=Vrefold;
end
 
Vrefold=Vref;
Vold=V;
Pold=P;
